simulink subsystem "AdjustEnvSustainParam"  (R2024a)
settings: Solver=VariableStepAuto  StartTime=0.0  StopTime=10.0  RelTol=1e-3
settings Model: Creator=david  LastModifiedBy=david

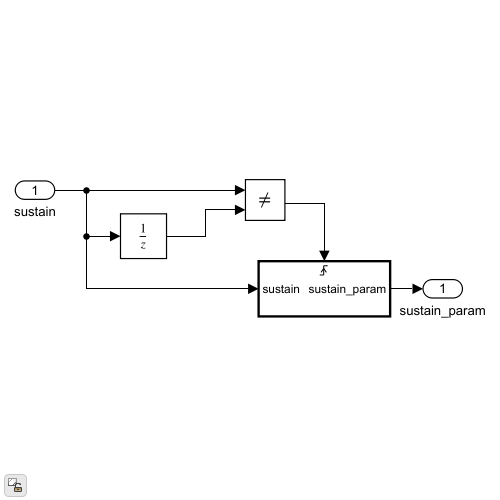
[thumbnail: Simulink's stored preview of the top-level diagram]
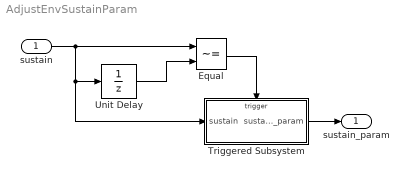
== system AdjustEnvSustainParam ==
  sustain : Inport
  Equal : RelationalOperator  Operator=~=  OutDataTypeStr=boolean  RndMeth=Simplest  InputSameDT=off
  Triggered Subsystem : Subsystem  TreatAsAtomicUnit=on
  Unit Delay : UnitDelay  SampleTime=-1  HasFrameUpgradeWarning=on
  sustain_param : Outport
  wires:
  sustain/1 -> Equal/1, Unit Delay/1, Triggered Subsystem/1(sustain)
  Unit Delay/1 -> Equal/2
  Equal/1 -> Triggered Subsystem/Trigger
  Triggered Subsystem/1(sustain_param) -> sustain_param/1

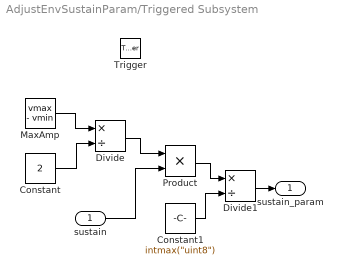
== system AdjustEnvSustainParam/Triggered Subsystem ==
  sustain : Inport
  Trigger : TriggerPort  VariantControl=(inherit)  InitialTriggerSignalState=zero
  Constant : Constant  Value=2  OutDataTypeStr=single
  Constant1 : Constant  Value="intmax(\"uint8\")"
  Divide : Product  Inputs=*/
  Divide1 : Product  Inputs=*/
  MaxAmp : Constant  Value=vmax - vmin
  Product : Product
  sustain_param : Outport
  wires:
  sustain/1 -> Product/2
  Divide1/1 -> sustain_param/1
  Constant/1 -> Divide/2
  Divide/1 -> Product/1
  MaxAmp/1 -> Divide/1
  Constant1/1 -> Divide1/2
  Product/1 -> Divide1/1
